simulink model "att1"  (R2018b)
settings: Solver=FixedStepAuto  StartTime=0.0  StopTime=10.0  FixedStep=dt  RelTol=1e-3
undefined symbols (not defined in the file or in its folder): GRAVITY_MSS, m
libraries: shared6dof x1, aerolibasang x1
settings Model: Creator=a4327  LastModifiedBy=a4327

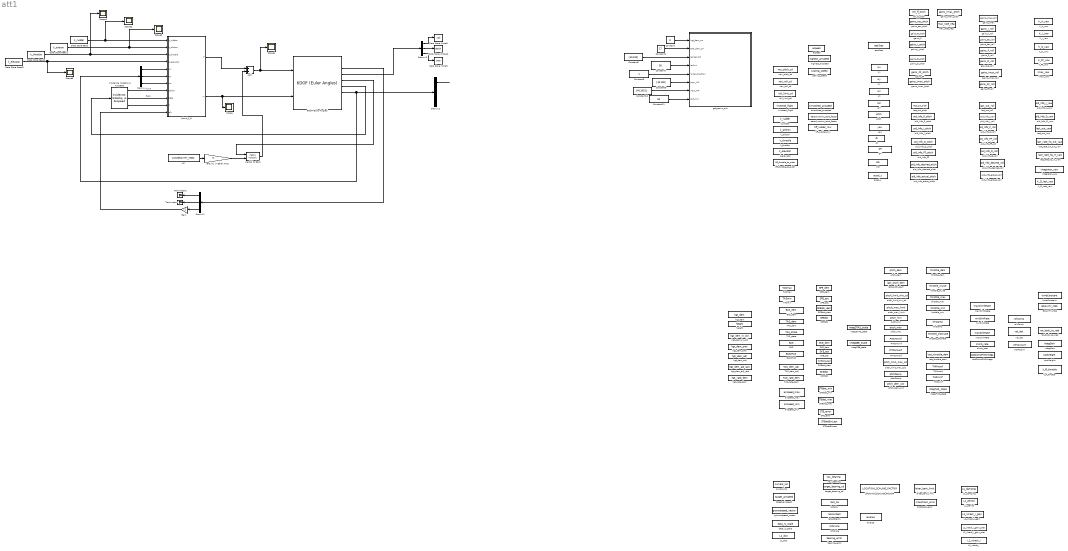
== system att1 ==
  6DOF (Euler Angles) : shared6dof/6DOF (Euler Angles)  units=Metric (MKS)  mtype=Fixed  rep=Euler Angles  xme_0=[0 0 0]  Vm_0=[17 0 0]  eul_0=[0 0 0]  pm_0=[0 0 0]  mass_0=m  mass_e=0.5  mass_f=2.0  inertia=J  inertia_e=eye(3)  inertia_f=2*eye(3)  k_quat=1.0  vre_flag=on  abi_flag=off  aMode=0  xme_statename=''  Vm_statename=''  eul_statename=''  quat_statename=''  pm_statename=''  mass_statename=''
      settings: SourceProductBaseCode=AE
  Add : Sum
  Constant : Constant  Value=0
  Constant1 : Constant  Value=17
  Constant10 : Constant  Value=[40,100.1]
  Constant11 : Constant  Value=50
  Constant6 : Constant  Value=[40,100]
  Constant7 : Constant  Value=50
  Constant8 : Constant
  Constant9 : Constant  Value=[40,100]
  DT : DataStoreMemory  DataStoreName=DT  ReadBeforeWriteMsg=warning  WriteAfterWriteMsg=warning  WriteAfterReadMsg=warning  InitialValue=DT  VectorParams1D=off  ShowAdditionalParam=off  OutDataTypeStr=double
  Data Store Read : DataStoreRead  DataStoreName=k_rudder
  Data Store Read1 : DataStoreRead  DataStoreName=k_aileron
  Data Store Read2 : DataStoreRead  DataStoreName=k_throttle
  Data Store Read3 : DataStoreRead  DataStoreName=k_elevator
  Data Store Write10 : DataStoreWrite  DataStoreName=pitch
  Data Store Write8 : DataStoreWrite  DataStoreName=roll
  Data Store Write9 : DataStoreWrite  DataStoreName=yaw
  Demux{,1..3} (4 alike) : Demux  Outputs=3
  EAS : DataStoreMemory  DataStoreName=EAS  ReadBeforeWriteMsg=warning  WriteAfterWriteMsg=warning  WriteAfterReadMsg=warning  InitialValue=EAS  VectorParams1D=off  ShowAdditionalParam=off  OutDataTypeStr=double
  EAS2TAS : DataStoreMemory  DataStoreName=EAS2TAS  ReadBeforeWriteMsg=warning  WriteAfterWriteMsg=warning  WriteAfterReadMsg=warning  InitialValue=EAS2TAS  VectorParams1D=off  ShowAdditionalParam=off  OutDataTypeStr=double
  EAS_dem : DataStoreMemory  DataStoreName=EAS_dem  ReadBeforeWriteMsg=warning  WriteAfterWriteMsg=warning  WriteAfterReadMsg=warning  InitialValue=EAS_dem  VectorParams1D=off  ShowAdditionalParam=off  OutDataTypeStr=double
  GRAVITY_MSS : DataStoreMemory  DataStoreName=GRAVITY_MSS  ReadBeforeWriteMsg=warning  WriteAfterWriteMsg=warning  WriteAfterReadMsg=warning  InitialValue=GRAVITY_MSS  VectorParams1D=off  ShowAdditionalParam=off  OutDataTypeStr=double
  Gain : Gain  Gain=-1
  Gravity in Earth Axes : Gain  Gain=m  SaturateOnIntegerOverflow=on  OutDataTypeStr=Inherit: Same as input  ParamDataTypeStr=Inherit: Same as input
  HD : DataStoreMemory  DataStoreName=HD  ReadBeforeWriteMsg=warning  WriteAfterWriteMsg=warning  WriteAfterReadMsg=warning  InitialValue=HD  ShowAdditionalParam=off  OutDataTypeStr=double
  "Incidence, Sideslip & Airspeed" : aerolibasang/Incidence, Sideslip, & Airspeed
      settings: SourceProductName=Aerospace Blockset
  Inertial to Body : Product  Multiplication=Matrix(*)  SaturateOnIntegerOverflow=on  InputSameDT=on  OutDataTypeStr=Inherit: Same as first input
  K_A_yaw : DataStoreMemory  DataStoreName=K_A_yaw  ReadBeforeWriteMsg=warning  WriteAfterWriteMsg=warning  WriteAfterReadMsg=warning  InitialValue=K_A_yaw  ShowAdditionalParam=off  OutDataTypeStr=double
  K_D_last_yaw : DataStoreMemory  DataStoreName=K_D_last_yaw  ReadBeforeWriteMsg=warning  WriteAfterWriteMsg=warning  WriteAfterReadMsg=warning  InitialValue=K_D_last_yaw  ShowAdditionalParam=off  OutDataTypeStr=double
  K_D_yaw : DataStoreMemory  DataStoreName=K_D_yaw  ReadBeforeWriteMsg=warning  WriteAfterWriteMsg=warning  WriteAfterReadMsg=warning  InitialValue=K_D_yaw  ShowAdditionalParam=off  OutDataTypeStr=double
  K_FF_yaw : DataStoreMemory  DataStoreName=K_FF_yaw  ReadBeforeWriteMsg=warning  WriteAfterWriteMsg=warning  WriteAfterReadMsg=warning  InitialValue=K_FF_yaw  ShowAdditionalParam=off  OutDataTypeStr=double
  K_I_yaw : DataStoreMemory  DataStoreName=K_I_yaw  ReadBeforeWriteMsg=warning  WriteAfterWriteMsg=warning  WriteAfterReadMsg=warning  InitialValue=K_I_yaw  ShowAdditionalParam=off  OutDataTypeStr=double
  L1_damping : DataStoreMemory  DataStoreName=L1_damping  ReadBeforeWriteMsg=warning  WriteAfterWriteMsg=warning  WriteAfterReadMsg=warning  InitialValue=L1_damping  VectorParams1D=off  ShowAdditionalParam=off  OutDataTypeStr=double
  L1_dist : DataStoreMemory  DataStoreName=L1_dist  ReadBeforeWriteMsg=warning  WriteAfterWriteMsg=warning  WriteAfterReadMsg=warning  InitialValue=L1_dist  VectorParams1D=off  ShowAdditionalParam=off  OutDataTypeStr=double
  L1_period : DataStoreMemory  DataStoreName=L1_period  ReadBeforeWriteMsg=warning  WriteAfterWriteMsg=warning  WriteAfterReadMsg=warning  InitialValue=L1_period  VectorParams1D=off  ShowAdditionalParam=off  OutDataTypeStr=double
  L1_xtrack_i : DataStoreMemory  DataStoreName=L1_xtrack_i  ReadBeforeWriteMsg=warning  WriteAfterWriteMsg=warning  WriteAfterReadMsg=warning  InitialValue=L1_xtrack_i  VectorParams1D=off  ShowAdditionalParam=off  OutDataTypeStr=double
  L1_xtrack_i_gain : DataStoreMemory  DataStoreName=L1_xtrack_i_gain  ReadBeforeWriteMsg=warning  WriteAfterWriteMsg=warning  WriteAfterReadMsg=warning  InitialValue=L1_xtrack_i_gain  VectorParams1D=off  ShowAdditionalParam=off  OutDataTypeStr=double
  L1_xtrack_i_gain_prev : DataStoreMemory  DataStoreName=L1_xtrack_i_gain_prev  ReadBeforeWriteMsg=warning  WriteAfterWriteMsg=warning  WriteAfterReadMsg=warning  InitialValue=L1_xtrack_i_gain_prev  VectorParams1D=off  ShowAdditionalParam=off  OutDataTypeStr=double
  LOCATION_SCALING_FACTOR : DataStoreMemory  DataStoreName=LOCATION_SCALING_FACTOR  ReadBeforeWriteMsg=warning  WriteAfterWriteMsg=warning  WriteAfterReadMsg=warning  InitialValue=LOCATION_SCALING_FACTOR  VectorParams1D=off  ShowAdditionalParam=off  OutDataTypeStr=double
  PITCHmaxf : DataStoreMemory  DataStoreName=PITCHmaxf  ReadBeforeWriteMsg=warning  WriteAfterWriteMsg=warning  WriteAfterReadMsg=warning  InitialValue=PITCHmaxf  VectorParams1D=off  ShowAdditionalParam=off  OutDataTypeStr=double
  PITCHminf : DataStoreMemory  DataStoreName=PITCHminf  ReadBeforeWriteMsg=warning  WriteAfterWriteMsg=warning  WriteAfterReadMsg=warning  InitialValue=PITCHminf  VectorParams1D=off  ShowAdditionalParam=off  OutDataTypeStr=double
  SKE_dem : DataStoreMemory  DataStoreName=SKE_dem  ReadBeforeWriteMsg=warning  WriteAfterWriteMsg=warning  WriteAfterReadMsg=warning  InitialValue=SKE_dem  VectorParams1D=off  ShowAdditionalParam=off  OutDataTypeStr=double
  SKE_est : DataStoreMemory  DataStoreName=SKE_est  ReadBeforeWriteMsg=warning  WriteAfterWriteMsg=warning  WriteAfterReadMsg=warning  InitialValue=SKE_est  VectorParams1D=off  ShowAdditionalParam=off  OutDataTypeStr=double
  SKEdot : DataStoreMemory  DataStoreName=SKEdot  ReadBeforeWriteMsg=warning  WriteAfterWriteMsg=warning  WriteAfterReadMsg=warning  InitialValue=SKEdot  VectorParams1D=off  ShowAdditionalParam=off  OutDataTypeStr=double
  SKEdot_dem : DataStoreMemory  DataStoreName=SKEdot_dem  ReadBeforeWriteMsg=warning  WriteAfterWriteMsg=warning  WriteAfterReadMsg=warning  InitialValue=SKEdot_dem  VectorParams1D=off  ShowAdditionalParam=off  OutDataTypeStr=double
  SPE_dem : DataStoreMemory  DataStoreName=SPE_dem  ReadBeforeWriteMsg=warning  WriteAfterWriteMsg=warning  WriteAfterReadMsg=warning  InitialValue=SPE_dem  VectorParams1D=off  ShowAdditionalParam=off  OutDataTypeStr=double
  SPE_est : DataStoreMemory  DataStoreName=SPE_est  ReadBeforeWriteMsg=warning  WriteAfterWriteMsg=warning  WriteAfterReadMsg=warning  InitialValue=SPE_est  VectorParams1D=off  ShowAdditionalParam=off  OutDataTypeStr=double
  SPEdot : DataStoreMemory  DataStoreName=SPEdot  ReadBeforeWriteMsg=warning  WriteAfterWriteMsg=warning  WriteAfterReadMsg=warning  InitialValue=SPEdot  VectorParams1D=off  ShowAdditionalParam=off  OutDataTypeStr=double
  SPEdot_dem : DataStoreMemory  DataStoreName=SPEdot_dem  ReadBeforeWriteMsg=warning  WriteAfterWriteMsg=warning  WriteAfterReadMsg=warning  InitialValue=SPEdot_dem  VectorParams1D=off  ShowAdditionalParam=off  OutDataTypeStr=double
  STE_error : DataStoreMemory  DataStoreName=STE_error  ReadBeforeWriteMsg=warning  WriteAfterWriteMsg=warning  WriteAfterReadMsg=warning  InitialValue=STE_error  VectorParams1D=off  ShowAdditionalParam=off  OutDataTypeStr=double
  STEdotErrLast : DataStoreMemory  DataStoreName=STEdotErrLast  ReadBeforeWriteMsg=warning  WriteAfterWriteMsg=warning  WriteAfterReadMsg=warning  InitialValue=STEdotErrLast  VectorParams1D=off  ShowAdditionalParam=off  OutDataTypeStr=double
  STEdot_max : DataStoreMemory  DataStoreName=STEdot_max  ReadBeforeWriteMsg=warning  WriteAfterWriteMsg=warning  WriteAfterReadMsg=warning  InitialValue=STEdot_max  VectorParams1D=off  ShowAdditionalParam=off  OutDataTypeStr=double
  STEdot_min : DataStoreMemory  DataStoreName=STEdot_min  ReadBeforeWriteMsg=warning  WriteAfterWriteMsg=warning  WriteAfterReadMsg=warning  InitialValue=STEdot_min  VectorParams1D=off  ShowAdditionalParam=off  OutDataTypeStr=double
  Scope{,1..5} (6 alike) : Scope
  TAS_dem : DataStoreMemory  DataStoreName=TAS_dem  ReadBeforeWriteMsg=warning  WriteAfterWriteMsg=warning  WriteAfterReadMsg=warning  InitialValue=TAS_dem  VectorParams1D=off  ShowAdditionalParam=off  OutDataTypeStr=double
  TAS_dem_adj : DataStoreMemory  DataStoreName=TAS_dem_adj  ReadBeforeWriteMsg=warning  WriteAfterWriteMsg=warning  WriteAfterReadMsg=warning  InitialValue=TAS_dem_adj  VectorParams1D=off  ShowAdditionalParam=off  OutDataTypeStr=double
  TAS_rate_dem : DataStoreMemory  DataStoreName=TAS_rate_dem  ReadBeforeWriteMsg=warning  WriteAfterWriteMsg=warning  WriteAfterReadMsg=warning  InitialValue=TAS_rate_dem  VectorParams1D=off  ShowAdditionalParam=off  OutDataTypeStr=double
  TAS_state : DataStoreMemory  DataStoreName=TAS_state  ReadBeforeWriteMsg=warning  WriteAfterWriteMsg=warning  WriteAfterReadMsg=warning  InitialValue=TAS_state  VectorParams1D=off  ShowAdditionalParam=off  OutDataTypeStr=double
  TASmax : DataStoreMemory  DataStoreName=TASmax  ReadBeforeWriteMsg=warning  WriteAfterWriteMsg=warning  WriteAfterReadMsg=warning  InitialValue=TASmax  VectorParams1D=off  ShowAdditionalParam=off  OutDataTypeStr=double
  TASmin : DataStoreMemory  DataStoreName=TASmin  ReadBeforeWriteMsg=warning  WriteAfterWriteMsg=warning  WriteAfterReadMsg=warning  InitialValue=TASmin  VectorParams1D=off  ShowAdditionalParam=off  OutDataTypeStr=double
  THRmaxf : DataStoreMemory  DataStoreName=THRmaxf  ReadBeforeWriteMsg=warning  WriteAfterWriteMsg=warning  WriteAfterReadMsg=warning  InitialValue=THRmaxf  VectorParams1D=off  ShowAdditionalParam=off  OutDataTypeStr=double
  THRminf : DataStoreMemory  DataStoreName=THRminf  ReadBeforeWriteMsg=warning  WriteAfterWriteMsg=warning  WriteAfterReadMsg=warning  InitialValue=THRminf  VectorParams1D=off  ShowAdditionalParam=off  OutDataTypeStr=double
  Terminator : Terminator
  Terminator1 : Terminator
  WPcircle : DataStoreMemory  DataStoreName=WPcircle  ReadBeforeWriteMsg=warning  WriteAfterWriteMsg=warning  WriteAfterReadMsg=warning  InitialValue=WPcircle  VectorParams1D=off  ShowAdditionalParam=off  OutDataTypeStr=double
  accel_y : DataStoreMemory  DataStoreName=accel_y  ReadBeforeWriteMsg=warning  WriteAfterWriteMsg=warning  WriteAfterReadMsg=warning  InitialValue=accel_y  ShowAdditionalParam=off  OutDataTypeStr=double
  aerodynamic_load_factor : DataStoreMemory  DataStoreName=aerodynamic_load_factor  ReadBeforeWriteMsg=warning  WriteAfterWriteMsg=warning  WriteAfterReadMsg=warning  InitialValue=aerodynamic_load_factor  ShowAdditionalParam=off  OutDataTypeStr=double
  airspeed_max : DataStoreMemory  DataStoreName=airspeed_max  ReadBeforeWriteMsg=warning  WriteAfterWriteMsg=warning  WriteAfterReadMsg=warning  InitialValue=airspeed_max  VectorParams1D=off  ShowAdditionalParam=off  OutDataTypeStr=double
  airspeed_min : DataStoreMemory  DataStoreName=airspeed_min  ReadBeforeWriteMsg=warning  WriteAfterWriteMsg=warning  WriteAfterReadMsg=warning  InitialValue=airspeed_min  VectorParams1D=off  ShowAdditionalParam=off  OutDataTypeStr=double
  aspeed : DataStoreMemory  DataStoreName=aspeed  ReadBeforeWriteMsg=warning  WriteAfterWriteMsg=warning  WriteAfterReadMsg=warning  InitialValue=aspeed  ShowAdditionalParam=off  OutDataTypeStr=double
  bearing_error : DataStoreMemory  DataStoreName=bearing_error  ReadBeforeWriteMsg=warning  WriteAfterWriteMsg=warning  WriteAfterReadMsg=warning  InitialValue=bearing_error  VectorParams1D=off  ShowAdditionalParam=off  OutDataTypeStr=double
  climb_rate : DataStoreMemory  DataStoreName=climb_rate  ReadBeforeWriteMsg=warning  WriteAfterWriteMsg=warning  WriteAfterReadMsg=warning  InitialValue=climb_rate  VectorParams1D=off  ShowAdditionalParam=off  OutDataTypeStr=double
  crosstrack_error : DataStoreMemory  DataStoreName=crosstrack_error  ReadBeforeWriteMsg=warning  WriteAfterWriteMsg=warning  WriteAfterReadMsg=warning  InitialValue=crosstrack_error  VectorParams1D=off  ShowAdditionalParam=off  OutDataTypeStr=double
  current_loc : DataStoreMemory  DataStoreName=current_loc  ReadBeforeWriteMsg=warning  WriteAfterWriteMsg=warning  WriteAfterReadMsg=warning  InitialValue=current_loc  VectorParams1D=off  ShowAdditionalParam=off  OutDataTypeStr=double
  data_is_stale : DataStoreMemory  DataStoreName=data_is_stale  ReadBeforeWriteMsg=warning  WriteAfterWriteMsg=warning  WriteAfterReadMsg=warning  InitialValue=data_is_stale  VectorParams1D=off  ShowAdditionalParam=off  OutDataTypeStr=double
  dt : DataStoreMemory  DataStoreName=dt  ReadBeforeWriteMsg=warning  WriteAfterWriteMsg=warning  WriteAfterReadMsg=warning  InitialValue=dt  ShowAdditionalParam=off  OutDataTypeStr=double
  eas2tas : DataStoreMemory  DataStoreName=eas2tas  ReadBeforeWriteMsg=warning  WriteAfterWriteMsg=warning  WriteAfterReadMsg=warning  InitialValue=eas2tas  ShowAdditionalParam=off  OutDataTypeStr=double
  gains_D_pitch : DataStoreMemory  DataStoreName=gains_D_pitch  ReadBeforeWriteMsg=warning  WriteAfterWriteMsg=warning  WriteAfterReadMsg=warning  InitialValue=gains_D_pitch  ShowAdditionalParam=off  OutDataTypeStr=double
  gains_D_roll : DataStoreMemory  DataStoreName=gains_D_roll  ReadBeforeWriteMsg=warning  WriteAfterWriteMsg=warning  WriteAfterReadMsg=warning  InitialValue=gains_D_roll  ShowAdditionalParam=off  OutDataTypeStr=double
  gains_FF : DataStoreMemory  DataStoreName=gains_FF_pitch  ReadBeforeWriteMsg=warning  WriteAfterWriteMsg=warning  WriteAfterReadMsg=warning  InitialValue=gains_FF_pitch  ShowAdditionalParam=off  OutDataTypeStr=double
  gains_FF_roll : DataStoreMemory  DataStoreName=gains_FF_roll  ReadBeforeWriteMsg=warning  WriteAfterWriteMsg=warning  WriteAfterReadMsg=warning  InitialValue=gains_FF_roll  ShowAdditionalParam=off  OutDataTypeStr=double
  gains_I_pitch : DataStoreMemory  DataStoreName=gains_I_pitch  ReadBeforeWriteMsg=warning  WriteAfterWriteMsg=warning  WriteAfterReadMsg=warning  InitialValue=gains_I_pitch  ShowAdditionalParam=off  OutDataTypeStr=double
  gains_I_roll : DataStoreMemory  DataStoreName=gains_I_roll  ReadBeforeWriteMsg=warning  WriteAfterWriteMsg=warning  WriteAfterReadMsg=warning  InitialValue=gains_I_roll  ShowAdditionalParam=off  OutDataTypeStr=double
  gains_P : DataStoreMemory  DataStoreName=gains_P_pitch  ReadBeforeWriteMsg=warning  WriteAfterWriteMsg=warning  WriteAfterReadMsg=warning  InitialValue=gains_P_pitch  ShowAdditionalParam=off  OutDataTypeStr=double
  gains_P_roll : DataStoreMemory  DataStoreName=gains_P_roll  ReadBeforeWriteMsg=warning  WriteAfterWriteMsg=warning  WriteAfterReadMsg=warning  InitialValue=gains_P_roll  ShowAdditionalParam=off  OutDataTypeStr=double
  gains_imax_pitch : DataStoreMemory  DataStoreName=gains_imax_pitch  ReadBeforeWriteMsg=warning  WriteAfterWriteMsg=warning  WriteAfterReadMsg=warning  InitialValue=gains_imax_pitch  ShowAdditionalParam=off  OutDataTypeStr=double
  gains_imax_roll : DataStoreMemory  DataStoreName=gains_imax_roll  ReadBeforeWriteMsg=warning  WriteAfterWriteMsg=warning  WriteAfterReadMsg=warning  InitialValue=gains_imax_roll  ShowAdditionalParam=off  OutDataTypeStr=double
  gains_rmax : DataStoreMemory  DataStoreName=gains_rmax_roll  ReadBeforeWriteMsg=warning  WriteAfterWriteMsg=warning  WriteAfterReadMsg=warning  InitialValue=gains_rmax_roll  ShowAdditionalParam=off  OutDataTypeStr=double
  gains_rmax_pitch : DataStoreMemory  DataStoreName=gains_rmax_pitch  ReadBeforeWriteMsg=warning  WriteAfterWriteMsg=warning  WriteAfterReadMsg=warning  InitialValue=gains_rmax_pitch  ShowAdditionalParam=off  OutDataTypeStr=double
  gains_tau_pitch : DataStoreMemory  DataStoreName=gains_tau_pitch  ReadBeforeWriteMsg=warning  WriteAfterWriteMsg=warning  WriteAfterReadMsg=warning  InitialValue=gains_tau_pitch  ShowAdditionalParam=off  OutDataTypeStr=double
  gains_tau_roll : DataStoreMemory  DataStoreName=gains_tau_roll  ReadBeforeWriteMsg=warning  WriteAfterWriteMsg=warning  WriteAfterReadMsg=warning  InitialValue=gains_tau_roll  ShowAdditionalParam=off  OutDataTypeStr=double
  get_servo_out : MATLAB Function  TreatAsAtomicUnit=on
  gn : Constant  Value=[0;0;GRAVITY_MSS]
  groundspeed_vector : DataStoreMemory  DataStoreName=groundspeed_vector  ReadBeforeWriteMsg=warning  WriteAfterWriteMsg=warning  WriteAfterReadMsg=warning  InitialValue=groundspeed_vector  VectorParams1D=off  ShowAdditionalParam=off  OutDataTypeStr=double
  height : DataStoreMemory  DataStoreName=height  ReadBeforeWriteMsg=warning  WriteAfterWriteMsg=warning  WriteAfterReadMsg=warning  InitialValue=height  VectorParams1D=off  ShowAdditionalParam=off  OutDataTypeStr=double
  hgt_dem : DataStoreMemory  DataStoreName=hgt_dem  ReadBeforeWriteMsg=warning  WriteAfterWriteMsg=warning  WriteAfterReadMsg=warning  InitialValue=hgt_dem  VectorParams1D=off  ShowAdditionalParam=off  OutDataTypeStr=double
  hgt_dem_adj : DataStoreMemory  DataStoreName=hgt_dem_adj  ReadBeforeWriteMsg=warning  WriteAfterWriteMsg=warning  WriteAfterReadMsg=warning  InitialValue=hgt_dem_adj  VectorParams1D=off  ShowAdditionalParam=off  OutDataTypeStr=double
  hgt_dem_adj_last : DataStoreMemory  DataStoreName=hgt_dem_adj_last  ReadBeforeWriteMsg=warning  WriteAfterWriteMsg=warning  WriteAfterReadMsg=warning  InitialValue=hgt_dem_adj_last  VectorParams1D=off  ShowAdditionalParam=off  OutDataTypeStr=double
  hgt_dem_in_old : DataStoreMemory  DataStoreName=hgt_dem_in_old  ReadBeforeWriteMsg=warning  WriteAfterWriteMsg=warning  WriteAfterReadMsg=warning  InitialValue=hgt_dem_in_old  VectorParams1D=off  ShowAdditionalParam=off  OutDataTypeStr=double
  hgt_dem_prev : DataStoreMemory  DataStoreName=hgt_dem_prev  ReadBeforeWriteMsg=warning  WriteAfterWriteMsg=warning  WriteAfterReadMsg=warning  InitialValue=hgt_dem_prev  VectorParams1D=off  ShowAdditionalParam=off  OutDataTypeStr=double
  hgt_rate_dem : DataStoreMemory  DataStoreName=hgt_rate_dem  ReadBeforeWriteMsg=warning  WriteAfterWriteMsg=warning  WriteAfterReadMsg=warning  InitialValue=hgt_rate_dem  VectorParams1D=off  ShowAdditionalParam=off  OutDataTypeStr=double
  highest_airspeed : DataStoreMemory  DataStoreName=highest_airspeed  ReadBeforeWriteMsg=warning  WriteAfterWriteMsg=warning  WriteAfterReadMsg=warning  InitialValue=highest_airspeed  ShowAdditionalParam=off  OutDataTypeStr=double
  imax_yaw : DataStoreMemory  DataStoreName=imax_yaw  ReadBeforeWriteMsg=warning  WriteAfterWriteMsg=warning  WriteAfterReadMsg=warning  InitialValue=imax_yaw  ShowAdditionalParam=off  OutDataTypeStr=double
  integDTAS_state : DataStoreMemory  DataStoreName=integDTAS_state  ReadBeforeWriteMsg=warning  WriteAfterWriteMsg=warning  WriteAfterReadMsg=warning  InitialValue=integDTAS_state  VectorParams1D=off  ShowAdditionalParam=off  OutDataTypeStr=double
  integGain : DataStoreMemory  DataStoreName=integGain  ReadBeforeWriteMsg=warning  WriteAfterWriteMsg=warning  WriteAfterReadMsg=warning  InitialValue=integGain  VectorParams1D=off  ShowAdditionalParam=off  OutDataTypeStr=double
  integSEB_state : DataStoreMemory  DataStoreName=integSEB_state  ReadBeforeWriteMsg=warning  WriteAfterWriteMsg=warning  WriteAfterReadMsg=warning  InitialValue=integSEB_state  VectorParams1D=off  ShowAdditionalParam=off  OutDataTypeStr=double
  integTHR_state : DataStoreMemory  DataStoreName=integTHR_state  ReadBeforeWriteMsg=warning  WriteAfterWriteMsg=warning  WriteAfterReadMsg=warning  InitialValue=integTHR_state  VectorParams1D=off  ShowAdditionalParam=off  OutDataTypeStr=double
  integrator_yaw : DataStoreMemory  DataStoreName=integrator_yaw  ReadBeforeWriteMsg=warning  WriteAfterWriteMsg=warning  WriteAfterReadMsg=warning  InitialValue=integrator_yaw  ShowAdditionalParam=off  OutDataTypeStr=double
  inverted_flight : DataStoreMemory  DataStoreName=inverted_flight  ReadBeforeWriteMsg=warning  WriteAfterWriteMsg=warning  WriteAfterReadMsg=warning  InitialValue=inverted_flight  ShowAdditionalParam=off  OutDataTypeStr=double
  k_aileron : DataStoreMemory  DataStoreName=k_aileron  ReadBeforeWriteMsg=warning  WriteAfterWriteMsg=warning  WriteAfterReadMsg=warning  InitialValue=k_aileron  ShowAdditionalParam=off  OutDataTypeStr=double
  k_elevator : DataStoreMemory  DataStoreName=k_elevator  ReadBeforeWriteMsg=warning  WriteAfterWriteMsg=warning  WriteAfterReadMsg=warning  InitialValue=k_elevator  ShowAdditionalParam=off  OutDataTypeStr=double
  k_ff_throttle : DataStoreMemory  DataStoreName=k_ff_throttle  ReadBeforeWriteMsg=warning  WriteAfterWriteMsg=warning  WriteAfterReadMsg=warning  InitialValue=k_ff_throttle  VectorParams1D=off  ShowAdditionalParam=off  OutDataTypeStr=double
  k_rudder : DataStoreMemory  DataStoreName=k_rudder  ReadBeforeWriteMsg=warning  WriteAfterWriteMsg=warning  WriteAfterReadMsg=warning  InitialValue=k_rudder  ShowAdditionalParam=off  OutDataTypeStr=double
  k_throttle : DataStoreMemory  DataStoreName=k_throttle  ReadBeforeWriteMsg=warning  WriteAfterWriteMsg=warning  WriteAfterReadMsg=warning  InitialValue=k_throttle  ShowAdditionalParam=off  OutDataTypeStr=double
  kff_rudder_mix : DataStoreMemory  DataStoreName=kff_rudder_mix  ReadBeforeWriteMsg=warning  WriteAfterWriteMsg=warning  WriteAfterReadMsg=warning  InitialValue=kff_rudder_mix  ShowAdditionalParam=off  OutDataTypeStr=double
  kff_throttle_to_pitch : DataStoreMemory  DataStoreName=kff_throttle_to_pitch  ReadBeforeWriteMsg=warning  WriteAfterWriteMsg=warning  WriteAfterReadMsg=warning  InitialValue=kff_throttle_to_pitch  ShowAdditionalParam=off  OutDataTypeStr=double
  last_Nu : DataStoreMemory  DataStoreName=last_Nu  ReadBeforeWriteMsg=warning  WriteAfterWriteMsg=warning  WriteAfterReadMsg=warning  InitialValue=last_Nu  VectorParams1D=off  ShowAdditionalParam=off  OutDataTypeStr=double
  last_out_pitch : DataStoreMemory  DataStoreName=last_out_pitch  ReadBeforeWriteMsg=warning  WriteAfterWriteMsg=warning  WriteAfterReadMsg=warning  InitialValue=last_out_pitch  ShowAdditionalParam=off  OutDataTypeStr=double
  last_out_roll : DataStoreMemory  DataStoreName=last_out_roll  ReadBeforeWriteMsg=warning  WriteAfterWriteMsg=warning  WriteAfterReadMsg=warning  InitialValue=last_out_roll  ShowAdditionalParam=off  OutDataTypeStr=double
  last_out_yaw : DataStoreMemory  DataStoreName=last_out_yaw  ReadBeforeWriteMsg=warning  WriteAfterWriteMsg=warning  WriteAfterReadMsg=warning  InitialValue=last_out_yaw  ShowAdditionalParam=off  OutDataTypeStr=double
  last_pitch_dem : DataStoreMemory  DataStoreName=last_pitch_dem  ReadBeforeWriteMsg=warning  WriteAfterWriteMsg=warning  WriteAfterReadMsg=warning  InitialValue=last_pitch_dem  VectorParams1D=off  ShowAdditionalParam=off  OutDataTypeStr=double
  last_rate_hp_in_yaw : DataStoreMemory  DataStoreName=last_rate_hp_in_yaw  ReadBeforeWriteMsg=warning  WriteAfterWriteMsg=warning  WriteAfterReadMsg=warning  InitialValue=last_rate_hp_in_yaw  ShowAdditionalParam=off  OutDataTypeStr=double
  last_rate_hp_out_yaw : DataStoreMemory  DataStoreName=last_rate_hp_out_yaw  ReadBeforeWriteMsg=warning  WriteAfterWriteMsg=warning  WriteAfterReadMsg=warning  InitialValue=last_rate_hp_out_yaw  ShowAdditionalParam=off  OutDataTypeStr=double
  last_throttle_dem : DataStoreMemory  DataStoreName=last_throttle_dem  ReadBeforeWriteMsg=warning  WriteAfterWriteMsg=warning  WriteAfterReadMsg=warning  InitialValue=last_throttle_dem  VectorParams1D=off  ShowAdditionalParam=off  OutDataTypeStr=double
  latAccDem1 : DataStoreMemory  DataStoreName=latAccDem  ReadBeforeWriteMsg=warning  WriteAfterWriteMsg=warning  WriteAfterReadMsg=warning  InitialValue=latAccDem  VectorParams1D=off  ShowAdditionalParam=off  OutDataTypeStr=double
  loiter_bank_limit : DataStoreMemory  DataStoreName=loiter_bank_limit  ReadBeforeWriteMsg=warning  WriteAfterWriteMsg=warning  WriteAfterReadMsg=warning  InitialValue=loiter_bank_limit  VectorParams1D=off  ShowAdditionalParam=off  OutDataTypeStr=double
  maxClimbRate : DataStoreMemory  DataStoreName=maxClimbRate  ReadBeforeWriteMsg=warning  WriteAfterWriteMsg=warning  WriteAfterReadMsg=warning  InitialValue=maxClimbRate  VectorParams1D=off  ShowAdditionalParam=off  OutDataTypeStr=double
  maxSinkRate : DataStoreMemory  DataStoreName=maxSinkRate  ReadBeforeWriteMsg=warning  WriteAfterWriteMsg=warning  WriteAfterReadMsg=warning  InitialValue=maxSinkRate  VectorParams1D=off  ShowAdditionalParam=off  OutDataTypeStr=double
  max_rate_neg : DataStoreMemory  DataStoreName=max_rate_neg  ReadBeforeWriteMsg=warning  WriteAfterWriteMsg=warning  WriteAfterReadMsg=warning  InitialValue=max_rate_neg  ShowAdditionalParam=off  OutDataTypeStr=double
  minSinkRate : DataStoreMemory  DataStoreName=minSinkRate  ReadBeforeWriteMsg=warning  WriteAfterWriteMsg=warning  WriteAfterReadMsg=warning  InitialValue=minSinkRate  VectorParams1D=off  ShowAdditionalParam=off  OutDataTypeStr=double
  nav_bearing : DataStoreMemory  DataStoreName=nav_bearing  ReadBeforeWriteMsg=warning  WriteAfterWriteMsg=warning  WriteAfterReadMsg=warning  InitialValue=nav_bearing  VectorParams1D=off  ShowAdditionalParam=off  OutDataTypeStr=double
  nav_pitch_cd : DataStoreMemory  DataStoreName=nav_pitch_cd  ReadBeforeWriteMsg=warning  WriteAfterWriteMsg=warning  WriteAfterReadMsg=warning  InitialValue=nav_pitch_cd  ShowAdditionalParam=off  OutDataTypeStr=double
  nav_roll_cd : DataStoreMemory  DataStoreName=nav_roll_cd  ReadBeforeWriteMsg=warning  WriteAfterWriteMsg=warning  WriteAfterReadMsg=warning  InitialValue=nav_roll_cd  ShowAdditionalParam=off  OutDataTypeStr=double
  pid_info_D_pitch : DataStoreMemory  DataStoreName=pid_info_D_pitch  ReadBeforeWriteMsg=warning  WriteAfterWriteMsg=warning  WriteAfterReadMsg=warning  InitialValue=pid_info_D_pitch  ShowAdditionalParam=off  OutDataTypeStr=double
  pid_info_D_roll : DataStoreMemory  DataStoreName=pid_info_D_roll  ReadBeforeWriteMsg=warning  WriteAfterWriteMsg=warning  WriteAfterReadMsg=warning  InitialValue=pid_info_D_roll  ShowAdditionalParam=off  OutDataTypeStr=double
  pid_info_D_yaw : DataStoreMemory  DataStoreName=pid_info_D_yaw  ReadBeforeWriteMsg=warning  WriteAfterWriteMsg=warning  WriteAfterReadMsg=warning  InitialValue=pid_info_D_yaw  ShowAdditionalParam=off  OutDataTypeStr=double
  pid_info_FF : DataStoreMemory  DataStoreName=pid_info_FF_pitch  ReadBeforeWriteMsg=warning  WriteAfterWriteMsg=warning  WriteAfterReadMsg=warning  InitialValue=pid_info_FF_pitch  ShowAdditionalParam=off  OutDataTypeStr=double
  pid_info_FF_roll : DataStoreMemory  DataStoreName=pid_info_FF_roll  ReadBeforeWriteMsg=warning  WriteAfterWriteMsg=warning  WriteAfterReadMsg=warning  InitialValue=pid_info_FF_roll  ShowAdditionalParam=off  OutDataTypeStr=double
  pid_info_I_pitch : DataStoreMemory  DataStoreName=pid_info_I_pitch  ReadBeforeWriteMsg=warning  WriteAfterWriteMsg=warning  WriteAfterReadMsg=warning  InitialValue=pid_info_I_pitch  ShowAdditionalParam=off  OutDataTypeStr=double
  pid_info_I_roll : DataStoreMemory  DataStoreName=pid_info_I_roll  ReadBeforeWriteMsg=warning  WriteAfterWriteMsg=warning  WriteAfterReadMsg=warning  InitialValue=pid_info_I_roll  ShowAdditionalParam=off  OutDataTypeStr=double
  pid_info_I_yaw : DataStoreMemory  DataStoreName=pid_info_I_yaw  ReadBeforeWriteMsg=warning  WriteAfterWriteMsg=warning  WriteAfterReadMsg=warning  InitialValue=pid_info_I_yaw  ShowAdditionalParam=off  OutDataTypeStr=double
  pid_info_P_pitch : DataStoreMemory  DataStoreName=pid_info_P_pitch  ReadBeforeWriteMsg=warning  WriteAfterWriteMsg=warning  WriteAfterReadMsg=warning  InitialValue=pid_info_P_pitch  ShowAdditionalParam=off  OutDataTypeStr=double
  pid_info_P_roll : DataStoreMemory  DataStoreName=pid_info_P_roll  ReadBeforeWriteMsg=warning  WriteAfterWriteMsg=warning  WriteAfterReadMsg=warning  InitialValue=pid_info_P_roll  ShowAdditionalParam=off  OutDataTypeStr=double
  pid_info_actua_pitchl : DataStoreMemory  DataStoreName=pid_info_actual_pitch  ReadBeforeWriteMsg=warning  WriteAfterWriteMsg=warning  WriteAfterReadMsg=warning  InitialValue=pid_info_actual_pitch  ShowAdditionalParam=off  OutDataTypeStr=double
  pid_info_actual_roll : DataStoreMemory  DataStoreName=pid_info_actual_roll  ReadBeforeWriteMsg=warning  WriteAfterWriteMsg=warning  WriteAfterReadMsg=warning  InitialValue=pid_info_actual_roll  ShowAdditionalParam=off  OutDataTypeStr=double
  pid_info_desired_pitch : DataStoreMemory  DataStoreName=pid_info_desired_pitch  ReadBeforeWriteMsg=warning  WriteAfterWriteMsg=warning  WriteAfterReadMsg=warning  InitialValue=pid_info_desired_pitch  ShowAdditionalParam=off  OutDataTypeStr=double
  pid_info_desired_roll : DataStoreMemory  DataStoreName=pid_info_desired_roll  ReadBeforeWriteMsg=warning  WriteAfterWriteMsg=warning  WriteAfterReadMsg=warning  InitialValue=pid_info_desired_roll  ShowAdditionalParam=off  OutDataTypeStr=double
  pitch : DataStoreMemory  DataStoreName=pitch  ReadBeforeWriteMsg=warning  WriteAfterWriteMsg=warning  WriteAfterReadMsg=warning  InitialValue=pitch  ShowAdditionalParam=off  OutDataTypeStr=double
  pitch_dem : DataStoreMemory  DataStoreName=pitch_dem  ReadBeforeWriteMsg=warning  WriteAfterWriteMsg=warning  WriteAfterReadMsg=warning  InitialValue=pitch_dem  VectorParams1D=off  ShowAdditionalParam=off  OutDataTypeStr=double
  pitch_dem_unc : DataStoreMemory  DataStoreName=pitch_dem_unc  ReadBeforeWriteMsg=warning  WriteAfterWriteMsg=warning  WriteAfterReadMsg=warning  InitialValue=pitch_dem_unc  VectorParams1D=off  ShowAdditionalParam=off  OutDataTypeStr=double
  pitch_limit_max_cd1 : DataStoreMemory  DataStoreName=pitch_limit_max_cd  ReadBeforeWriteMsg=warning  WriteAfterWriteMsg=warning  WriteAfterReadMsg=warning  InitialValue=pitch_limit_max_cd  VectorParams1D=off  ShowAdditionalParam=off  OutDataTypeStr=double
  pitch_limit_min_cd : DataStoreMemory  DataStoreName=pitch_limit_min_cd  ReadBeforeWriteMsg=warning  WriteAfterWriteMsg=warning  WriteAfterReadMsg=warning  InitialValue=pitch_limit_min_cd  VectorParams1D=off  ShowAdditionalParam=off  OutDataTypeStr=double
  pitch_max : DataStoreMemory  DataStoreName=pitch_max  ReadBeforeWriteMsg=warning  WriteAfterWriteMsg=warning  WriteAfterReadMsg=warning  InitialValue=pitch_max  VectorParams1D=off  ShowAdditionalParam=off  OutDataTypeStr=double
  pitch_max_limit : DataStoreMemory  DataStoreName=pitch_max_limit  ReadBeforeWriteMsg=warning  WriteAfterWriteMsg=warning  WriteAfterReadMsg=warning  InitialValue=pitch_max_limit  VectorParams1D=off  ShowAdditionalParam=off  OutDataTypeStr=double
  pitch_min : DataStoreMemory  DataStoreName=pitch_min  ReadBeforeWriteMsg=warning  WriteAfterWriteMsg=warning  WriteAfterReadMsg=warning  InitialValue=pitch_min  VectorParams1D=off  ShowAdditionalParam=off  OutDataTypeStr=double
  pland_F_M : MATLAB Function  TreatAsAtomicUnit=on
  ptchDamp : DataStoreMemory  DataStoreName=ptchDamp  ReadBeforeWriteMsg=warning  WriteAfterWriteMsg=warning  WriteAfterReadMsg=warning  InitialValue=ptchDamp  VectorParams1D=off  ShowAdditionalParam=off  OutDataTypeStr=double
  reverse : DataStoreMemory  DataStoreName=reverse  ReadBeforeWriteMsg=warning  WriteAfterWriteMsg=warning  WriteAfterReadMsg=warning  InitialValue=reverse  VectorParams1D=off  ShowAdditionalParam=off  OutDataTypeStr=double
  roll : DataStoreMemory  DataStoreName=roll  ReadBeforeWriteMsg=warning  WriteAfterWriteMsg=warning  WriteAfterReadMsg=warning  InitialValue=roll  ShowAdditionalParam=off  OutDataTypeStr=double
  rollComp : DataStoreMemory  DataStoreName=rollComp  ReadBeforeWriteMsg=warning  WriteAfterWriteMsg=warning  WriteAfterReadMsg=warning  InitialValue=rollComp  VectorParams1D=off  ShowAdditionalParam=off  OutDataTypeStr=double
  roll_ff_pitch : DataStoreMemory  DataStoreName=roll_ff_pitch  ReadBeforeWriteMsg=warning  WriteAfterWriteMsg=warning  WriteAfterReadMsg=warning  InitialValue=roll_ff_pitch  ShowAdditionalParam=off  OutDataTypeStr=double
  roll_limit_cd : DataStoreMemory  DataStoreName=roll_limit_cd  ReadBeforeWriteMsg=warning  WriteAfterWriteMsg=warning  WriteAfterReadMsg=warning  InitialValue=roll_limit_cd  ShowAdditionalParam=off  OutDataTypeStr=double
  rot_body_to_ned : DataStoreMemory  DataStoreName=rot_body_to_ned  ReadBeforeWriteMsg=warning  WriteAfterWriteMsg=warning  WriteAfterReadMsg=warning  InitialValue=rot_body_to_ned  VectorParams1D=off  ShowAdditionalParam=off  OutDataTypeStr=double
  scaling_speed : DataStoreMemory  DataStoreName=scaling_speed  ReadBeforeWriteMsg=warning  WriteAfterWriteMsg=warning  WriteAfterReadMsg=warning  InitialValue=scaling_speed  ShowAdditionalParam=off  OutDataTypeStr=double
  smoothed_airspeed : DataStoreMemory  DataStoreName=smoothed_airspeed  ReadBeforeWriteMsg=warning  WriteAfterWriteMsg=warning  WriteAfterReadMsg=warning  InitialValue=smoothed_airspeed  ShowAdditionalParam=off  OutDataTypeStr=double
  spdCompFiltOmega : DataStoreMemory  DataStoreName=spdCompFiltOmega  ReadBeforeWriteMsg=warning  WriteAfterWriteMsg=warning  WriteAfterReadMsg=warning  InitialValue=spdCompFiltOmega  VectorParams1D=off  ShowAdditionalParam=off  OutDataTypeStr=double
  spdWeight : DataStoreMemory  DataStoreName=spdWeight  ReadBeforeWriteMsg=warning  WriteAfterWriteMsg=warning  WriteAfterReadMsg=warning  InitialValue=spdWeight  VectorParams1D=off  ShowAdditionalParam=off  OutDataTypeStr=double
  target_airspeed : DataStoreMemory  DataStoreName=target_airspeed  ReadBeforeWriteMsg=warning  WriteAfterWriteMsg=warning  WriteAfterReadMsg=warning  InitialValue=target_airspeed  VectorParams1D=off  ShowAdditionalParam=off  OutDataTypeStr=double
  target_bearing_cd : DataStoreMemory  DataStoreName=target_bearing_cd  ReadBeforeWriteMsg=warning  WriteAfterWriteMsg=warning  WriteAfterReadMsg=warning  InitialValue=target_bearing_cd  VectorParams1D=off  ShowAdditionalParam=off  OutDataTypeStr=double
  thrDamp : DataStoreMemory  DataStoreName=thrDamp  ReadBeforeWriteMsg=warning  WriteAfterWriteMsg=warning  WriteAfterReadMsg=warning  InitialValue=thrDamp  VectorParams1D=off  ShowAdditionalParam=off  OutDataTypeStr=double
  throttle_cruise : DataStoreMemory  DataStoreName=throttle_cruise  ReadBeforeWriteMsg=warning  WriteAfterWriteMsg=warning  WriteAfterReadMsg=warning  InitialValue=throttle_cruise  VectorParams1D=off  ShowAdditionalParam=off  OutDataTypeStr=double
  throttle_dem : DataStoreMemory  DataStoreName=throttle_dem  ReadBeforeWriteMsg=warning  WriteAfterWriteMsg=warning  WriteAfterReadMsg=warning  InitialValue=throttle_dem  VectorParams1D=off  ShowAdditionalParam=off  OutDataTypeStr=double
  throttle_max : DataStoreMemory  DataStoreName=throttle_max  ReadBeforeWriteMsg=warning  WriteAfterWriteMsg=warning  WriteAfterReadMsg=warning  InitialValue=throttle_max  VectorParams1D=off  ShowAdditionalParam=off  OutDataTypeStr=double
  throttle_min : DataStoreMemory  DataStoreName=throttle_min  ReadBeforeWriteMsg=warning  WriteAfterWriteMsg=warning  WriteAfterReadMsg=warning  InitialValue=throttle_min  VectorParams1D=off  ShowAdditionalParam=off  OutDataTypeStr=double
  throttle_slewrate : DataStoreMemory  DataStoreName=throttle_slewrate  ReadBeforeWriteMsg=warning  WriteAfterWriteMsg=warning  WriteAfterReadMsg=warning  InitialValue=throttle_slewrate  VectorParams1D=off  ShowAdditionalParam=off  OutDataTypeStr=double
  timeConstant : DataStoreMemory  DataStoreName=timeConstant  ReadBeforeWriteMsg=warning  WriteAfterWriteMsg=warning  WriteAfterReadMsg=warning  InitialValue=timeConstant  VectorParams1D=off  ShowAdditionalParam=off  OutDataTypeStr=double
  vel_dot : DataStoreMemory  DataStoreName=vel_dot  ReadBeforeWriteMsg=warning  WriteAfterWriteMsg=warning  WriteAfterReadMsg=warning  InitialValue=vel_dot  VectorParams1D=off  ShowAdditionalParam=off  OutDataTypeStr=double
  vertAccLim : DataStoreMemory  DataStoreName=vertAccLim  ReadBeforeWriteMsg=warning  WriteAfterWriteMsg=warning  WriteAfterReadMsg=warning  InitialValue=vertAccLim  VectorParams1D=off  ShowAdditionalParam=off  OutDataTypeStr=double
  wx : DataStoreMemory  DataStoreName=wx  ReadBeforeWriteMsg=warning  WriteAfterWriteMsg=warning  WriteAfterReadMsg=warning  InitialValue=wx  ShowAdditionalParam=off  OutDataTypeStr=double
  wy : DataStoreMemory  DataStoreName=wy  ReadBeforeWriteMsg=warning  WriteAfterWriteMsg=warning  WriteAfterReadMsg=warning  InitialValue=wy  ShowAdditionalParam=off  OutDataTypeStr=double
  wz : DataStoreMemory  DataStoreName=wz  ReadBeforeWriteMsg=warning  WriteAfterWriteMsg=warning  WriteAfterReadMsg=warning  InitialValue=wz  ShowAdditionalParam=off  OutDataTypeStr=double
  yaw : DataStoreMemory  DataStoreName=yaw  ReadBeforeWriteMsg=warning  WriteAfterWriteMsg=warning  WriteAfterReadMsg=warning  InitialValue=yaw  VectorParams1D=off  ShowAdditionalParam=off  OutDataTypeStr=double
  wires:
  Constant9/1 -> get_servo_out/6(prev_WP)
  Constant8/1 -> get_servo_out/5(loiter_direction)
  Constant6/1 -> get_servo_out/3(center_WP)
  Constant10/1 -> get_servo_out/7(next_WP)
  Constant11/1 -> get_servo_out/8(dist_min)
  Constant7/1 -> get_servo_out/4(radius)
  Demux/1 -> pland_F_M/5(wx)
  Demux/3 -> pland_F_M/7(wz)
  pland_F_M/2(M) -> Scope/1, 6DOF (Euler Angles)/2
  gn/1 -> Gravity in Earth Axes/1
  Data Store Read2/1 -> Scope4/1, pland_F_M/3(k_throttle)
  Inertial to Body/1 -> Add/2
  6DOF (Euler Angles)/5 -> "Incidence, Sideslip & Airspeed"/1
  Demux/2 -> pland_F_M/6(wy)
  6DOF (Euler Angles)/6 -> Demux2/1, Demux/1
  Gravity in Earth Axes/1 -> Inertial to Body/2
  pland_F_M/1(F) -> Add/1
  Data Store Read1/1 -> Scope3/1, pland_F_M/2(k_aileron)
  Add/1 -> Scope1/1, 6DOF (Euler Angles)/1
  Data Store Read/1 -> Scope2/1, pland_F_M/1(k_rudder)
  6DOF (Euler Angles)/4 -> Inertial to Body/1
  "Incidence, Sideslip & Airspeed"/1 -> pland_F_M/8(alpha)  "Alpha"
  "Incidence, Sideslip & Airspeed"/3 -> pland_F_M/10(V)
  "Incidence, Sideslip & Airspeed"/2 -> pland_F_M/9(beta)  "Beta"
  6DOF (Euler Angles)/2 -> Demux1/1
  Demux1/2 -> Terminator/1
  Demux1/1 -> Terminator1/1
  Demux1/3 -> Gain/1
  Gain/1 -> pland_F_M/11(alt)
  Data Store Read3/1 -> pland_F_M/4(k_elevator), Scope5/1
  Constant/1 -> get_servo_out/1(hgt_dem_cm)
  Constant1/1 -> get_servo_out/2(EAS_dem_cm)
  Demux2/1 -> ?
  Demux3/2 -> Data Store Write10/1
  Demux3/1 -> Data Store Write8/1
  Demux3/3 -> Data Store Write9/1
  6DOF (Euler Angles)/3 -> Demux3/1

== matlab function att1/get_servo_out ==
  data: dt data_store_memory; wy data_store_memory; gains_I_pitch data_store_memory; gains_tau_pitch data_store_memory; gains_P_pitch data_store_memory; gains_D_pitch data_store_memory; gains_imax_pitch data_store_memory; gains_FF_pitch data_store_memory; airspeed_min data_store_memory; last_out_pitch data_store_memory; pid_info_I_pitch data_store_memory; pid_info_P_pitch data_store_memory; pid_info_FF_pitch data_store_memory; pid_info_D_pitch data_store_memory; pid_info_desired_pitch data_store_memory; pid_info_actual_pitch data_store_memory; eas2tas data_store_memory; roll data_store_memory; pitch data_store_memory; roll_limit_cd data_store_memory; aspeed data_store_memory; max_rate_neg data_store_memory; gains_rmax_pitch data_store_memory; GRAVITY_MSS data_store_memory; roll_ff_pitch data_store_memory; HD data_store_memory; gains_D_roll data_store_memory; gains_FF_roll data_store_memory; gains_I_roll data_store_memory; gains_imax_roll data_store_memory; gains_P_roll data_store_memory; gains_rmax_roll data_store_memory; gains_tau_roll data_store_memory; last_out_roll data_store_memory; pid_info_actual_roll data_store_memory; pid_info_D_roll data_store_memory; pid_info_desired_roll data_store_memory; pid_info_FF_roll data_store_memory; pid_info_I_roll data_store_memory; pid_info_P_roll data_store_memory; wx data_store_memory; accel_y data_store_memory; imax_yaw data_store_memory; integrator_yaw data_store_memory; K_A_yaw data_store_memory; K_D_last_yaw data_store_memory; K_D_yaw data_store_memory; K_FF_yaw data_store_memory; K_I_yaw data_store_memory; last_out_yaw data_store_memory; last_rate_hp_in_yaw data_store_memory; last_rate_hp_out_yaw data_store_memory; pid_info_D_yaw data_store_memory; pid_info_I_yaw data_store_memory; wz data_store_memory; throttle_dem data_store_memory; pitch_dem data_store_memory; pitch_limit_min_cd data_store_memory; pitch_limit_max_cd data_store_memory; nav_pitch_cd data_store_memory; nav_roll_cd data_store_memory; inverted_flight data_store_memory; k_rudder data_store_memory; k_aileron data_store_memory; k_throttle data_store_memory; k_elevator data_store_memory; kff_throttle_to_pitch data_store_memory; highest_airspeed data_store_memory; scaling_speed data_store_memory; airspeed_max data_store_memory; latAccDem data_store_memory; smoothed_airspeed data_store_memory; aerodynamic_load_factor data_store_memory; kff_rudder_mix data_store_memory; hgt_dem_cm input; EAS_dem_cm input; TASmax data_store_memory; SKE_dem data_store_memory; TASmin data_store_memory; SPE_dem data_store_memory; SPE_est data_store_memory; SKE_est data_store_memory; STE_error data_store_memory; SPEdot_dem data_store_memory; SKEdot_dem data_store_memory; STEdot_min data_store_memory; STEdot_max data_store_memory; SPEdot data_store_memory; SKEdot data_store_memory; STEdotErrLast data_store_memory; timeConstant data_store_memory; throttle_cruise data_store_memory; rot_body_to_ned data_store_memory; rollComp data_store_memory; THRmaxf data_store_memory; THRminf data_store_memory; thrDamp data_store_memory; throttle_slewrate data_store_memory; last_throttle_dem data_store_memory; DT data_store_memory; integGain data_store_memory; integTHR_state data_store_memory; maxClimbRate data_store_memory; minSinkRate data_store_memory; EAS_dem data_store_memory; hgt_dem data_store_memory; throttle_max data_store_memory; throttle_min data_store_memory; pitch_max data_store_memory; PITCHmaxf data_store_memory; pitch_min data_store_memory; PITCHminf data_store_memory; pitch_max_limit data_store_memory; TAS_dem data_store_memory; EAS2TAS data_store_memory; EAS data_store_memory; TAS_state data_store_memory; integDTAS_state data_store_memory; spdCompFiltOmega data_store_memory; vel_dot data_store_memory; TAS_dem_adj data_store_memory; TAS_rate_dem data_store_memory; hgt_dem_in_old data_store_memory; maxSinkRate data_store_memory; hgt_dem_prev data_store_memory; hgt_dem_adj_last data_store_memory; hgt_dem_adj data_store_memory; hgt_rate_dem data_store_memory; height data_store_memory; climb_rate data_store_memory; spdWeight data_store_memory; ptchDamp data_store_memory; pitch_dem_unc data_store_memory; integSEB_state data_store_memory; vertAccLim data_store_memory; last_pitch_dem data_store_memory; k_ff_throttle data_store_memory; center_WP input; radius input; loiter_direction input; prev_WP input; next_WP input; dist_min input; L1_damping data_store_memory; L1_period data_store_memory; current_loc data_store_memory; groundspeed_vector data_store_memory; target_bearing_cd data_store_memory; L1_dist data_store_memory; crosstrack_error data_store_memory; nav_bearing data_store_memory; L1_xtrack_i_gain data_store_memory; L1_xtrack_i_gain_prev data_store_memory; L1_xtrack_i data_store_memory; last_Nu data_store_memory; WPcircle data_store_memory; data_is_stale data_store_memory; bearing_error data_store_memory; LOCATION_SCALING_FACTOR data_store_memory; yaw data_store_memory; reverse data_store_memory; loiter_bank_limit data_store_memory; target_airspeed data_store_memory
function get_servo_out(   hgt_dem_cm, EAS_dem_cm, center_WP,   radius,   loiter_direction,prev_WP,  next_WP,  dist_min)
global aerodynamic_load_factor
% update_pitch_throttle(  hgt_dem_cm,EAS_dem_cm,aerodynamic_load_factor)
% update_loiter( center_WP,   radius,   loiter_direction)
% update_waypoint( prev_WP,  next_WP,  dist_min)
calc_nav_pitch();
calc_nav_roll()
calc_throttle()
stabilize()

== matlab function att1/pland_F_M ==
  data: F output; k_rudder input; k_aileron input; k_throttle input; k_elevator input; wx input; wy input; wz input; alpha input; beta input; V input; alt input; M output
function [F,M]   = pland_F_M(k_rudder,k_aileron,k_throttle,k_elevator,wx,wy,wz,alpha,beta,V,alt)
    
%推力模型，Thr=throttle_dem*Tmax，throttle_dem=24N。
%阻力模型，Cx_Sref=Cx_Sref_alpha*alpha,Cx_Sref_alpha=0.007;
%升力模型  Cy_Sref=Cy_Sref_alpha*(alpha0+alpha),Cy_Sref_alpha=0.022,alpha0=5;
Tmax=36;

% Sref=0.3;

Cx_Sref_alpha=0.0215;%50/155/15
Cz_Sref_alpha=0.1075;
HD=180/pi;
alpha0=3/HD;

Cx_Sref=Cx_Sref_alpha;
Cz_Sref=Cz_Sref_alpha*(alpha+alpha0)*HD;
Cy=0;

[~,~,rho,~] = atom_mode(alt);
q=0.5*rho*V*V;
L=-q*Cz_Sref;
D=-q*Cx_Sref+k_throttle*Tmax;
C=0;
% F=[L ];

F=[D C L];
%%%%%%%%%%%%%%%%%%%%%%%%%%%
dmya=-0.2549;  %(2*pi*1.5)^2*Jy/HD
dmye=dmya/2;
dmy_wy=0.1;
%%%%%%%%%%%%%%%%%%%%%%%%%
dmxa=12.8312;    %(2*pi*10)^2*Jx/HD
dmx_wx=0.1;


Mx=dmxa*k_aileron/100-dmx_wx*wx;
My=dmye*k_elevator/100+dmya*alpha-dmy_wy*wy;
Mz=0;

M=[Mx; My ;Mz];
end
